simulink model "tanks"  (R2021a)
settings: Solver=VariableStepAuto  StartTime=0.0  StopTime=200  RelTol=1e-3  EnableMultiTasking=on
libraries: nesl_utility x5, fl_lib x3, sh_lib x3, adrc_toolbox_library x2
settings Model: Creator=johnh  LastModifiedBy=krzysztof
settings SolverCC: AlgebraicLoopSolver=TrustRegion
settings OptimizationCC: LifeSpan=inf
settings DebuggingCC: SFUnexpectedBacktrackingDiag=warning  SFNoUnconditionalDefaultTransitionDiag=warning  SFExecutionAtInitializationDiag=none  SFMachineParentedDataDiag=warning  ArithmeticOperatorsInVariantConditions=warning
settings SFSimCC: SimUseLocalCustomCode=off  CustomCodeUndefinedFunction=UseInterfaceOnly
settings RTWCC: RTWUseLocalCustomCode=off
settings CodeAppCC: StateflowObjectComments=on
settings GRTTargetCC: TargetLangStandard=C89/C90 (ANSI)
settings ConfigComp: CovMetricSettings=dw  CovSaveCumulativeToWorkspaceVar=on  CovSaveSingleToWorkspaceVar=on  CovExternalEMLEnable=off

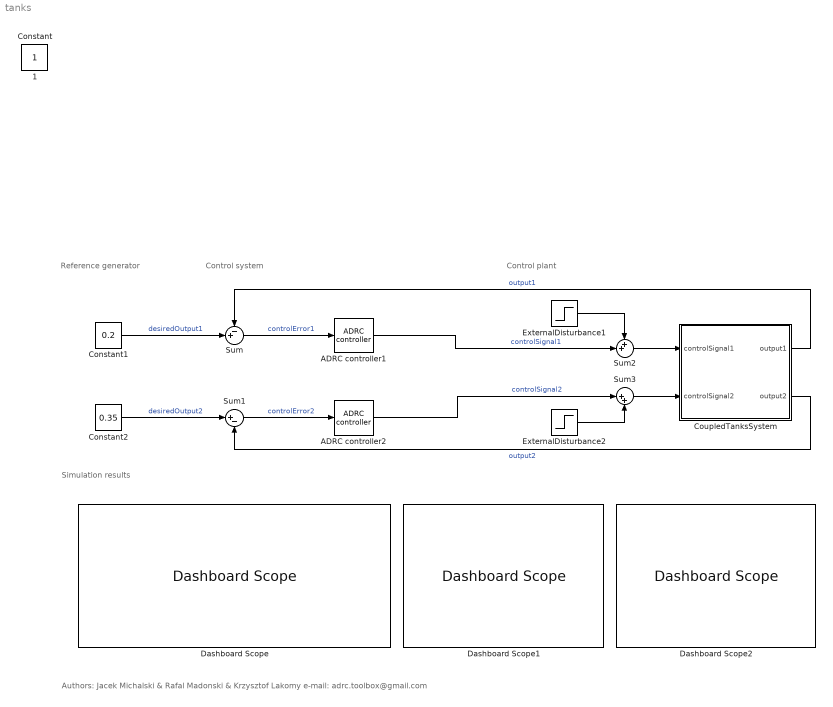
== system tanks ==
  note: Authors: Jacek Michalski & Rafal Madonski & Krzysztof Lakomy
      | e-mail: adrc.toolbox@gmail.com
  note: Simulation results
  note: Control system
  note: Control plant
  note: Reference
      | generator
  ADRC controller1 : adrc_toolbox_library/ADRC controller  dynamicsOrder=2  inputGainParameter=0.8  inputGainSource=Internal  observerBandwidth=3  observerBandwidthSource=Internal  controllerBandwidth=0.3  controllerBandwidthSource=Internal  saturationEnabled=on  UpperLimit=4e-4  LowerLimit=0  deadTimeEnabled=off  deadTime=0.2  observerOutputEnabled=off  observerOutputChoice=Estimated total disturbance
      settings: SourceProductName=ADRC toolbox
  ADRC controller2 : adrc_toolbox_library/ADRC controller  dynamicsOrder=2  inputGainParameter=1  inputGainSource=Internal  observerBandwidth=1.2  observerBandwidthSource=Internal  controllerBandwidth=0.12  controllerBandwidthSource=Internal  saturationEnabled=on  UpperLimit=4e-4  LowerLimit=0  deadTimeEnabled=off  deadTime=0.2  observerOutputEnabled=off  observerOutputChoice=Estimated total disturbance
      settings: SourceProductName=ADRC toolbox
  Constant1 : Constant  Value=0.2  SampleTime=-1
  Constant2 : Constant  Value=0.35  SampleTime=-1
  CoupledTanksSystem : Subsystem
      mask Display: image('$imagefile'); % Use "Edit Image" on toolstrip to change.
  Dashboard Scope : DashboardScope  Ymin=0  Ymax=100
  Dashboard Scope1 : DashboardScope  Ymin=0  Ymax=100
  Dashboard Scope2 : DashboardScope  Ymin=-50  Ymax=50
  ExternalDisturbance1 : Step  Time=90  After=-1.4e-4  SampleTime=0
  ExternalDisturbance2 : Step  Time=130  After=-0.7e-4  SampleTime=0
  Sum : Sum  Inputs=-+|
  Sum1 : Sum  Inputs=|+-
  Sum2 : Sum  Inputs=++|
  Sum3 : Sum  Inputs=|++
  1 : Constant  IOType=siggen
  Constant : Constant  IOType=siggen
  wires:
  CoupledTanksSystem/1(output1) -> Sum/1  "output1"
  Constant1/1 -> Sum/2  "desiredOutput1"
  Sum/1 -> ADRC controller1/1  "controlError1"
  ADRC controller2/1 -> Sum3/1  "controlSignal2"
  Sum1/1 -> ADRC controller2/1  "controlError2"
  Constant2/1 -> Sum1/1  "desiredOutput2"
  CoupledTanksSystem/2(output2) -> Sum1/2  "output2"
  ADRC controller1/1 -> Sum2/2  "controlSignal1"
  ExternalDisturbance1/1 -> Sum2/1
  ExternalDisturbance2/1 -> Sum3/2
  Sum2/1 -> CoupledTanksSystem/1(controlSignal1)
  Sum3/1 -> CoupledTanksSystem/2("controlSignal2 ")

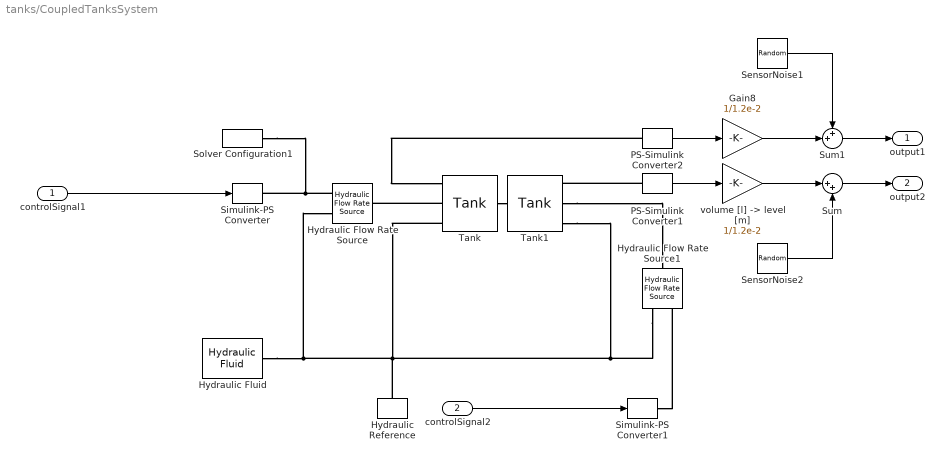
== system tanks/CoupledTanksSystem ==
  controlSignal1 : Inport
  "controlSignal2 " : Inport  Port=2
  Gain8 : Gain  Gain=1/1.2e-2
  Hydraulic Flow Rate Source : fl_lib/Hydraulic/Hydraulic Sources/Hydraulic Flow Rate Source
      settings: SourceProductBaseCode=SS  InternalSimscapePortConfiguration="{\"Bottom\":[],\"Left\":[{\"id\":\"P\",\"label\":\"P\",\"type\":\"foundation.hydraulic.hydraulic\"}],\"Right\":[{\"id\":\"S\",\"label\":\"S\",\"type\":\"input\"},{\"id\":\"T\",\"label\":\"T\",\"type\":\"foundation.hydraulic.hydraulic\"}],\"Top\":[]}"
  Hydraulic Flow Rate Source1 : fl_lib/Hydraulic/Hydraulic Sources/Hydraulic Flow Rate Source
      settings: SourceProductBaseCode=SS  InternalSimscapePortConfiguration="{\"Bottom\":[],\"Left\":[{\"id\":\"P\",\"label\":\"P\",\"type\":\"foundation.hydraulic.hydraulic\"}],\"Right\":[{\"id\":\"S\",\"label\":\"S\",\"type\":\"input\"},{\"id\":\"T\",\"label\":\"T\",\"type\":\"foundation.hydraulic.hydraulic\"}],\"Top\":[]}"
  Hydraulic Fluid : sh_lib/Hydraulic Utilities/Hydraulic Fluid  DataSource=1  SelFluid=24  SysTemp=60  TrapAir=0.005  ViscDerFactor=1  range_error=1
  Hydraulic Reference : fl_lib/Hydraulic/Hydraulic Elements/Hydraulic Reference
  PS-Simulink Converter1 : nesl_utility/PS-Simulink Converter  PhysicalDomain=network_engine_domain  SubClassName=ps_output  LeftPortType=input  RightPortType=output  PseudoPeriodic=off  Frequencies=[]  Unit=1  AffineConversion=off
      settings: SourceProductBaseCode=PW,SS
  PS-Simulink Converter2 : nesl_utility/PS-Simulink Converter  PhysicalDomain=network_engine_domain  SubClassName=ps_output  LeftPortType=input  RightPortType=output  PseudoPeriodic=off  Frequencies=[]  Unit=1  AffineConversion=off
      settings: SourceProductBaseCode=PW,SS
  SensorNoise1 : RandomNumber  Variance=0.8e-10  SampleTime=0.1
  SensorNoise2 : RandomNumber  Variance=0.8e-10  SampleTime=0.1
  Simulink-PS Converter : nesl_utility/Simulink-PS Converter  PhysicalDomain=network_engine_domain  SubClassName=ps_input  LeftPortType=input  RightPortType=output  PseudoPeriodic=off  Frequencies=[]  NoiseDistribution=none  NoiseParameters=[]  Unit=1  AffineConversion=off  FilteringAndDerivatives=provide  SimscapeFilterOrder=1  InputFilterTimeConstant=0.001  UdotUserProvided=0
      settings: SourceProductBaseCode=PW,SS
  Simulink-PS Converter1 : nesl_utility/Simulink-PS Converter  PhysicalDomain=network_engine_domain  SubClassName=ps_input  LeftPortType=input  RightPortType=output  PseudoPeriodic=off  Frequencies=[]  NoiseDistribution=none  NoiseParameters=[]  Unit=1  AffineConversion=off  FilteringAndDerivatives=provide  SimscapeFilterOrder=1  InputFilterTimeConstant=0.001  UdotUserProvided=0
      settings: SourceProductBaseCode=PW,SS
  Solver Configuration1 : nesl_utility/Solver Configuration  PhysicalDomain=network_engine_domain  SubClassName=solver  LeftPortType=input  RightPortType=generic  Tones=[]  Harmonics=[]  SimulateNoise=off  Profile=off  UseLocalSampling=off  EnableSwitchedLinearOptims=on  FrequencyDomain=off  UseCCode=off  RelTol=0.001  AbsTol=1e-06  MinStep=1e-09  ToWorkspace=off  RevertToSquareIcSolve=off  NumHomotopyIterations=100  PhasorMode=off  PhasorModeNumHarmonics=1  DoDC=off  ResidualTolerance=1e-09  UseLocalSolver=off  LocalSolverChoice=NE_BACKWARD_EULER_ADVANCER  LocalSolverSampleTime=0.001  DoFixedCost=off  MaxNonlinIter=3  MaxModeIter=2  ComputeImpulses=off  ImpulseIterations=2  LinearAlgebra=Full  EquationFormulation=NE_TIME_EF  DelaysMemoryBudget=1024  AutomaticFiltering=on  FilteringTimeConstant=0.001  PartitionStorageMethod=AS_NEEDED  PartitionMemoryBudget=1024  PartitionMethod=FAST
      settings: SourceProductBaseCode=PW,SS
  Sum : Sum  Inputs=|++
  Sum1 : Sum  Inputs=++|
  Tank : sh_lib/Low-Pressure Blocks/Tank  press=0 Pa  level_spec=1  tank_area=1.2e-2 m^2  fluid_volume_tab=[0, .0028, .0065, .0114, .0176, .0252, .0344, .0436, .0512, .0574, .0623, .066, .0688, .0707, .072, .0727] m^3  fluid_level_tab=[0, .02, .04, .06, .08, .1, .12, .14, .16, .18, .2, .22, .24, .26, .28, .3] m  interp_method=1  extrap_method=2  pipe_diam=0.02 cm  loss_coeff=1.2  g=9.80665 m/s^2  min_level=1e-3 cm  fluid_level_check=0  volume_specify=on  volume_priority=High  volume=0 l  volume_nominal_specify=off  volume_nominal_unit=l  volume_nominal_value=1  level_specify=on  level_priority=None  level=0 m  level_nominal_specify=off  level_nominal_unit=m  level_nominal_value=1  pipe_diam_A=(4*7.5e-5/pi)^0.5 m  loss_coeff_A=1.2  height_B=0.8 m  pipe_diam_B=(4*7.5e-5/pi)^0.5 m  loss_coeff_B=1.2  height_C=0.0 m  pipe_diam_C=(4*7.5e-5/pi)^0.5 m  loss_coeff_C=1.2
      settings: SourceProductBaseCode=SH  InternalSimscapePortConfiguration="{\"Bottom\":[],\"Left\":[{\"id\":\"V\",\"label\":\"V\",\"type\":\"output\"},{\"id\":\"B\",\"label\":\"B\",\"type\":\"foundation.hydraulic.hydraulic\"},{\"id\":\"A\",\"label\":\"A\",\"type\":\"foundation.hydraulic.hydraulic\"}],\"Right\":[{\"id\":\"C\",\"label\":\"C\",\"type\":\"foundation.hydraulic.hydraulic\"}],\"Top\":[]}"
  Tank1 : sh_lib/Low-Pressure Blocks/Tank  press=0 Pa  level_spec=1  tank_area=1.2e-2 m^2  fluid_volume_tab=[0, .0028, .0065, .0114, .0176, .0252, .0344, .0436, .0512, .0574, .0623, .066, .0688, .0707, .072, .0727] m^3  fluid_level_tab=[0, .02, .04, .06, .08, .1, .12, .14, .16, .18, .2, .22, .24, .26, .28, .3] m  interp_method=1  extrap_method=1  pipe_diam=0.02 cm  loss_coeff=1.2  g=9.80665 m/s^2  min_level=1e-3 cm  fluid_level_check=0  volume_specify=on  volume_priority=High  volume=0 l  volume_nominal_specify=off  volume_nominal_unit=l  volume_nominal_value=1  level_specify=on  level_priority=None  level=0 m  level_nominal_specify=off  level_nominal_unit=m  level_nominal_value=1  pipe_diam_A=(4*7.5e-5/pi)^0.5 m  loss_coeff_A=1.2  height_B=0.8 m  pipe_diam_B=(4*7.5e-5/pi)^0.5 m  loss_coeff_B=1.2  height_C=0.0 m  pipe_diam_C=(4*7.5e-5/pi)^0.5 m  loss_coeff_C=1.2
      settings: SourceProductBaseCode=SH  InternalSimscapePortConfiguration="{\"Bottom\":[],\"Left\":[{\"id\":\"V\",\"label\":\"V\",\"type\":\"output\"},{\"id\":\"B\",\"label\":\"B\",\"type\":\"foundation.hydraulic.hydraulic\"},{\"id\":\"A\",\"label\":\"A\",\"type\":\"foundation.hydraulic.hydraulic\"}],\"Right\":[{\"id\":\"C\",\"label\":\"C\",\"type\":\"foundation.hydraulic.hydraulic\"}],\"Top\":[]}"
  "volume [l] -> level [m]" : Gain  Gain=1/1.2e-2
  output1 : Outport  VectorParamsAs1DForOutWhenUnconnected=off
  output2 : Outport  Port=2  VectorParamsAs1DForOutWhenUnconnected=off
  wires:
  PS-Simulink Converter2/1 -> Gain8/1
  PS-Simulink Converter1/1 -> "volume [l] -> level [m]"/1
  controlSignal1/1 -> Simulink-PS Converter/1
  "controlSignal2 "/1 -> Simulink-PS Converter1/1
  Gain8/1 -> Sum1/2
  "volume [l] -> level [m]"/1 -> Sum/1
  SensorNoise1/1 -> Sum1/1
  SensorNoise2/1 -> Sum/2
  Sum/1 -> output2/1
  Sum1/1 -> output1/1
  connections:
  Hydraulic Flow Rate Source1/RConn2 -- Tank1/LConn3 -- Tank/LConn3 -- Hydraulic Reference/LConn1 -- Hydraulic Flow Rate Source/RConn2 -- Hydraulic Fluid/RConn1
  Hydraulic Flow Rate Source/RConn1 -- Simulink-PS Converter/RConn1 -- Solver Configuration1/RConn1
  Tank/LConn2 -- Hydraulic Flow Rate Source/LConn1
  PS-Simulink Converter1/LConn1 -- Tank1/LConn1
  Tank/RConn1 -- Tank1/RConn1
  PS-Simulink Converter2/LConn1 -- Tank/LConn1
  Tank1/LConn2 -- Hydraulic Flow Rate Source1/LConn1
  Simulink-PS Converter1/RConn1 -- Hydraulic Flow Rate Source1/RConn1
